simulink model "bike_model"  (R2018b)
settings: Solver=ode23s  StartTime=0.0  StopTime=sim_time  FixedStep=Ts_IMU  MaxStep=Ts  RelTol=1e-3
values from neighbouring files (symbols this model uses):
  a_compFilter = b_compFilter - 0.77    (= 0.325)    [configuration.m]
  A_kalman = [1 0 Ts 0; 0 1 0 Ts; 0 0 1 0; 0 0 0 1]    [configuration.m]
  b_compFilter = 1.095    [configuration.m]
  B_kalman = [0 0 0 0; 0 0 0 0; 0 0 0 0; 0 0 0 0]    [configuration.m]
  b_real = 1.095    [configuration.m]
  C_kalman = [1 0 0 0; 0 1 0 0; 0 0 1 0; 0 0 0 1]    [configuration.m]
  complementary = 0.985    [configuration.m]
  D_kalman = [0 0 0 0; 0 0 0 0; 0 0 0 0; 0 0 0 0]    [configuration.m]
  damp = 0.4    [configuration.m]
  Dead_Band = [0.055, -0.055, 0.005]    [configuration.m]
  delay = 0.045    [configuration.m]
  direct_control = 1    [configuration.m]
  filter_model = 1    [configuration.m]
  forward_motor_dynamics = 0    [configuration.m]
  fr_oscil = 1    [configuration.m]
  g = 9.81    [configuration.m]
  gain = 0.3    [configuration.m]
  I_direct = 0.000227125326188444    (= 0.000227125326188)    [configuration.m]
  I_lat = 0.000115580509653549    (= 0.000115580509654)    [configuration.m]
  I_steer = 0.4510120195392    (= 0.451012019539)    [configuration.m]
  IMU_height_model = 0.45    [configuration.m]
  IMU_height_real = 0.45    [configuration.m]
  initial_states = [deg2rad(-2) deg2rad(0) deg2rad(0)]    [configuration.m]
  input_velocity = 3    [configuration.m]
  lambda_compFilter = deg2rad(70)    [configuration.m]
  lambda_real = deg2rad(70)    [configuration.m]
  lat_control = 1    [configuration.m]
  look_ahead = 0    [configuration.m]
  max_handlebar = 40*(pi/180)    (= 0.698131700798)    [configuration.m]
  max_roll = pi/2    (= 1.57079632679)    [configuration.m]
  max_steering_motor_acc = inf    [configuration.m]
  max_steering_motor_speed = 7.5    [configuration.m]
  min_handlebar = -max_handlebar    (= -0.698131700798)    [configuration.m]
  min_roll = - max_roll    (= -1.57079632679)    [configuration.m]
  min_steering_motor_acc = -inf    [configuration.m]
  min_steering_motor_speed = -7.5    [configuration.m]
  noise = 0    [configuration.m]
  noise_acc = 2.4869e-05    [configuration.m]
  noise_encoder = 1e-7    (= 1e-07)    [configuration.m]
  noise_gyro = 0.0022    [configuration.m]
  noise_hall = 0    [configuration.m]
  noise_pos_meas = 0.51    [configuration.m]
  osc_roll = 0    [configuration.m]
  osc_steer = 0    [configuration.m]
  P_direct = 0.0712859744206787    (= 0.0712859744207)    [configuration.m]
  P_lat = 0.0465435246389258    (= 0.0465435246389)    [configuration.m]
  P_steer = 0.219020351848633    (= 0.219020351849)    [configuration.m]
  parameters_compFilter = [g h_compFilter b_compFilter a_compFilter lambda_compFilter c_compFilter]    [configuration.m]
  parameters_f_b_real = [m_frame_real m_box_real h_frame_real h_box_real a_frame_real a_box_real c_frame_real c_box_real b_frame_real b_box_real l_frame_real l_box_real]    [configuration.m]
  parameters_real = [g h_real b_real a_real lambda_real c_real]    [configuration.m]
  path_tracking = 1    [configuration.m]
  plant_model = 1    [configuration.m]
  R_kalman = [noise_pos_meas 0 0 0; 0 noise_pos_meas 0 0; 0 0 noise_hall 0; 0 0 0 noise_hall]    [configuration.m]
  roll_rate_coef = 0.9    [configuration.m]
  steer_control = 1    [configuration.m]
  steering_motor_limitations = 0    [configuration.m]
  Ts = 0.04    [configuration.m]
  Ts_IMU = 0.04    [configuration.m]
undefined symbols (not defined in the file or in its folder): A, B, cumulative_dist_along_path, curvature, Discrete, initial_x, initial_y, lqr_gains, path_x, path_y, sys_con, sys_dis, Time, velocity_lqr
libraries: simulink x22, simulink_extras x2, dspsigops x2, ctrlSharedLib x1
(part 3 of 3)

== system bike_model/Complementary filter/Roll Angle Estimation of Accelerometer/Lateral Acceleration Compensator/Subsystem ==
  In1 : Inport
  Constant : Constant  Value=A
  Constant1 : Constant  Value=B
  Delay1 : Delay  DelayLength=1  InitialCondition=[0 0 0]  SampleTime=Ts_IMU
  Multiply : Product  Multiplication=Matrix(*)
  Multiply1 : Product  Multiplication=Matrix(*)
  Sum2 : Sum  Inputs=|++
  Out1 : Outport
  wires:
  Sum2/1 -> Delay1/1
  Multiply1/1 -> Sum2/2
  In1/1 -> Multiply1/2  "u"
  Delay1/1 -> Multiply/2, Out1/1  "x"
  Multiply/1 -> Sum2/1
  Constant/1 -> Multiply/1
  Constant1/1 -> Multiply1/1

== matlab function bike_model/Balance Controller/Reference States/Reference Roll Angle Calculator ==
  data: parameters_real input; velocity input; delta_ref input; phi_ref output
function phi_ref = fcn(parameters_real, velocity, delta_ref)
g = parameters_real(1);
b = parameters_real(3);
v = velocity;

phi_ref = -atan(v^2 / (g * b) * delta_ref); % tan(theta_ref));

== matlab function bike_model/Physical Bike/Linear Bicycle Model ==
  data: states input; input input; xdot output; velocity input; disturbance input; parameters_real input; parameters_f_b_real input
function xdot = fcn(states,input,velocity,disturbance,parameters_real,parameters_f_b_real)

delta_d=input;
v=velocity;
d1=disturbance(1);
d2=disturbance(2);
d3=disturbance(3);

% 1=frame | 2=box
m1=parameters_f_b_real(1);
m2=parameters_f_b_real(2);
h1=parameters_f_b_real(3);
h2=parameters_f_b_real(4);
a1=parameters_f_b_real(5);
a2=parameters_f_b_real(6);
c1=parameters_f_b_real(7);
c2=parameters_f_b_real(8);
b1=parameters_f_b_real(9);
b2=parameters_f_b_real(10);
l1=parameters_f_b_real(11);
l2=parameters_f_b_real(12);

g=parameters_real(1);
%h=parameters_real(2);
b=parameters_real(3);
%a=parameters_real(4);
lambda=parameters_real(5);
c=parameters_real(6);

phi=states(1);
delta=states(2);
phi_d=states(3);

A=((m1/12)*((c1^2)+(b1^2)))+(m1*(h1^2))+((m2/12)*((c2^2)+(b2^2)))+(m2*(h2^2));
B=((m1/12)*((l1^2)+(b1^2)))-(m1*a1*h1)+((m2/12)*((c2^2)+(b2^2)))+(m2*a2*h2);
D=(((m1*h1)+(m2*h2))*(v^2))-(c*g*((m1*a1)-(m2*a2)));

xdot1=phi_d+d1;
xdot2=delta_d+d2;
xdot3=((((m1*h1)+(m2*h2))*g)/A)*phi+((D*sin(lambda))/(b*A))*delta+d3+((B*v*sin(lambda))/(b*A))*delta_d;

xdot=[xdot1 xdot2 xdot3];

== matlab function bike_model/Global Angles and Coordinates Calculator - Position/Measured Bike Angles to Global Angles/MATLAB Function ==
  data: v input; parameters_model input; delta input; psi_d output; beta output
function [psi_d, beta]  = fcn(v, parameters_model, delta)

b = parameters_model(3);
a = parameters_model(4);

beta = atan((a / (b)) * tan(delta));
psi_d = (v / a) * sin(beta);

== matlab function bike_model/Reference Position /Variable Look Ahead/Look-Ahead Coefficient Modifier (Slow Turn-Off)  ==
  data: look_ahead input; look_ahead_modified output; feedback input; time input; time_delayed input
function look_ahead_modified = fcn(look_ahead, feedback, time, time_delayed)

step=time-time_delayed;

kill_time=3;

delta=(feedback*step)/kill_time;

if look_ahead-feedback<-0.0001
    look_ahead_modified=feedback-delta;
else
    look_ahead_modified = look_ahead;
end
    

end

== matlab function bike_model/Global Angles and Coordinates Calculator - Position/Measured Global Angles to Global Coordinates/MATLAB Function1 ==
  data: v input; psi input; Xdot output; beta input; Ydot output
function [Xdot, Ydot]  = fcn(v, psi, beta)

Xdot = v * cos(psi + beta);
Ydot = v * sin(psi + beta);

== matlab function bike_model/Reference Position /Variable Look Ahead/Look-Ahead Coefficient Selector ==
  data: curv_next input; look_ahead output; curv input
function look_ahead = fcn(curv_next, curv)


if curv>-0.01 && curv<0.01
    curv=0;
end

if curv_next>-0.01 && curv_next<0.01
    curv_next=0;
end



if curv>=0
    if curv-curv_next>0
        look_ahead=0;
    else
        look_ahead=curv_next-curv;
    end
else
    if curv-curv_next<0
        look_ahead=0;
    else
        look_ahead=curv-curv_next;
    end
end



end

== matlab function bike_model/Complementary filter/Roll Angle Estimation of Accelerometer/Lateral Acceleration Compensator/Linear Bicycle Model ==
  data: states input; input input; xdot output; velocity input; parameters_model input
function xdot = fcn(states,input,velocity,parameters_model)

delta_d=input;
v=velocity;

g=parameters_model(1);
h=parameters_model(2);
b=parameters_model(3);
a=parameters_model(4);
lambda=parameters_model(5);
c=parameters_model(6);

phi=states(1);
delta=states(2);
phi_d=states(3);

xdot1=phi_d;
xdot2=delta_d;
xdot3=(g/h)*phi+((a*v)/(b*h))*sin(lambda)*delta_d+((h*v^2-g*a*c)/(b*h^2))*sin(lambda)*delta;

xdot=[xdot1 xdot2 xdot3];

== matlab function bike_model/Physical Bike/Global Angles and Coordinates Calculator - Position/Measured Bike Angles to Global Angles/MATLAB Function ==
  data: v input; parameters_model input; delta input; psi_d output; beta output
function [psi_d, beta]  = fcn(v, parameters_model, delta)

b = parameters_model(3);
a = parameters_model(4);

beta = atan((a / (b)) * tan(delta));
psi_d = (v / a) * sin(beta);

== matlab function bike_model/Physical Bike/Nonlinear Bicycle Model ==
  data: states input; input input; xdot output; velocity input; disturbance input; parameters_real input; parameters_f_b_real input
function xdot = fcn(states,input,velocity,disturbance,parameters_real,parameters_f_b_real)

delta_d=input;
v=velocity;
d1=disturbance(1);
d2=disturbance(2);
d3=disturbance(3);

% 1=frame | 2=box
m1=parameters_f_b_real(1);
m2=parameters_f_b_real(2);
h1=parameters_f_b_real(3);
h2=parameters_f_b_real(4);
a1=parameters_f_b_real(5);
a2=parameters_f_b_real(6);
c1=parameters_f_b_real(7);
c2=parameters_f_b_real(8);
b1=parameters_f_b_real(9);
b2=parameters_f_b_real(10);
l1=parameters_f_b_real(11);
l2=parameters_f_b_real(12);

g=parameters_real(1);
%h=parameters_real(2);
b=parameters_real(3);
%a=parameters_real(4);
lambda=parameters_real(5);
c=parameters_real(6);

A=((m1/12)*((c1^2)+(b1^2)))+(m1*(h1^2))+((m2/12)*((c2^2)+(b2^2)))+(m2*(h2^2));
B=(m1*a1*h1)-(m2*a2*h2);
D=(((m1*h1)+(m2*h2))*(v^2))-(c*g*((m1*a1)-(m2*a2)));

phi=states(1);
delta=states(2);
phi_d=states(3);

% Biaised mass from box mass measurement
m = 9.3;
d = 0.03;
T = m*d*g*cos(phi)/A;
T = 0;

% Biaised mass from bike equilibrium measurement
% m = 9.3;
% d = 0.07;
% T = m*d*g*cos(phi)/A;
% % T = 0;

xdot1=phi_d+d1;
xdot2=delta_d+d2;
xdot3=((((m1*h1)+(m2*h2))*g)/A)*tan(phi) + T +((D*sin(lambda))/(b*A))*tan(delta)+d3+((B*v*sin(lambda))/(b*A))*tan(delta_d);

xdot=[xdot1 xdot2 xdot3];

== matlab function bike_model/Physical Bike/Linear Bicycle Model with neglected fork angle (lambda=90deg, c=0) "THE SIMPLEST MODEL" ==
  data: states input; input input; xdot output; velocity input; disturbance input; parameters_real input; parameters_f_b_real input
function xdot = fcn(states,input,velocity,disturbance,parameters_real,parameters_f_b_real)

delta_d=input;
v=velocity;
d1=disturbance(1);
d2=disturbance(2);
d3=disturbance(3);

% 1=frame | 2=box
m1=parameters_f_b_real(1);
m2=parameters_f_b_real(2);
h1=parameters_f_b_real(3);
h2=parameters_f_b_real(4);
a1=parameters_f_b_real(5);
a2=parameters_f_b_real(6);
c1=parameters_f_b_real(7);
c2=parameters_f_b_real(8);
b1=parameters_f_b_real(9);
b2=parameters_f_b_real(10);
l1=parameters_f_b_real(11);
l2=parameters_f_b_real(12);

g=parameters_real(1);
%h=parameters_real(2);
b=parameters_real(3);
%a=parameters_real(4);
lambda=parameters_real(5);
c=parameters_real(6);

A=((m1/12)*((c1^2)+(b1^2)))+(m1*(h1^2))+((m2/12)*((c2^2)+(b2^2)))+(m2*(h2^2));
B=((m1/12)*((l1^2)+(b1^2)))-(m1*a1*h1)+((m2/12)*((c2^2)+(b2^2)))+(m2*a2*h2);
D=(((m1*h1)+(m2*h2))*(v^2))-(c*g*((m1*a1)-(m2*a2)));

phi=states(1);
delta=states(2);
phi_d=states(3);

xdot1=phi_d+d1;
xdot2=delta_d+d2;
xdot3=((((m1*h1)+(m2*h2))*g)/A)*phi+((D*sin(lambda))/(b*A))*delta+d3+((B*v*sin(lambda))/(b*A))*delta_d;

xdot=[xdot1 xdot2 xdot3];

== matlab function bike_model/Global Angles and Coordinates Calculator - Velocity/Measured Bike Angles to Global Angles/MATLAB Function ==
  data: v input; parameters_model input; delta input; psi_d output; beta output
function [psi_d, beta]  = fcn(v, parameters_model, delta)

b = parameters_model(3);
a = parameters_model(4);

beta = atan((a / (b)) * tan(delta));
psi_d = (v / a) * sin(beta);

== matlab function bike_model/Complementary filter/Roll Angle Estimation of Accelerometer/Lateral Acceleration Compensator/Linear Bicycle Model1 ==
  data: states input; input input; xdot output; velocity input; parameters_model input
function xdot = fcn(states,input,velocity,parameters_model)

delta_d=input;
v=velocity;

g=parameters_model(1);
h=parameters_model(2);
b=parameters_model(3);
a=parameters_model(4);
lambda=parameters_model(5);
c=parameters_model(6);

phi=states(1);
delta=states(2);
phi_d=states(3);

xdot1=phi_d;
xdot2=delta_d;
xdot3=(g/h)*phi+((a*v)/(b*h))*sin(lambda)*delta_d+((h*v^2-g*a*c)/(b*h^2))*sin(lambda)*delta;

xdot=[xdot1; xdot2; xdot3];

== matlab function bike_model/Complementary filter/Roll Angle Estimation of Accelerometer/Lateral Acceleration Compensator/discrete ==
  data: states input; input input; x_next output; A input; B input
function x_next = fcn(states,input,A,B)





x_next=A*states+B*input;

== matlab function bike_model/Global Angles and Coordinates Calculator - Velocity/Measured Global Angles to Global Coordinates/MATLAB Function1 ==
  data: v input; psi input; Xdot output; beta input; Ydot output
function [Xdot, Ydot]  = fcn(v, psi, beta)

Xdot = v * cos(psi + beta);
Ydot = v * sin(psi + beta);

== matlab function bike_model/Physical Bike/Global Angles and Coordinates Calculator - Position/Measured Global Angles to Global Coordinates/MATLAB Function1 ==
  data: v input; psi input; Xdot output; beta input; Ydot output
function [Xdot, Ydot]  = fcn(v, psi, beta)

Xdot = v * cos(psi + beta);
Ydot = v * sin(psi + beta);
